simulink model "pratica_3_c"  (R2021a)
settings: Solver=VariableStepAuto  StartTime=0.0  StopTime=2  RelTol=1e-3
undefined symbols (not defined in the file): DiscIntNeverNeededParam
settings Model: Creator=ribeiro  LastModifiedBy=ribeiro

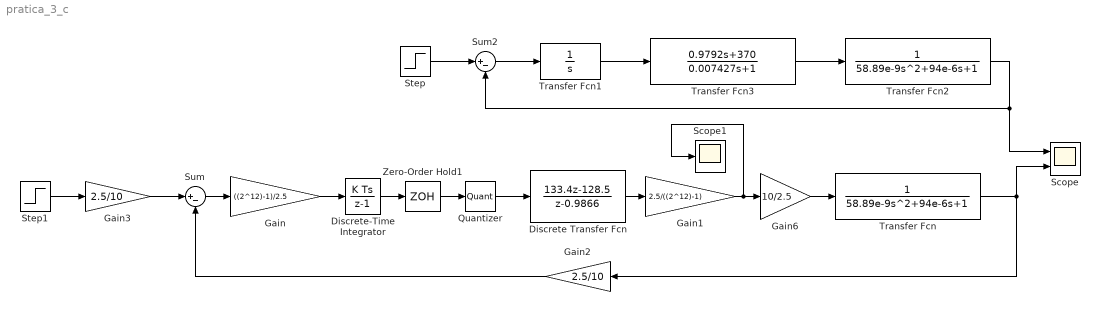
== system pratica_3_c ==
  Discrete Transfer Fcn : DiscreteTransferFcn  Numerator=[133.4 -128.5]  Denominator=[1 -0.9866]
  Discrete-Time Integrator : DiscreteIntegrator  SampleTime=-1  ICPrevOutput=DiscIntNeverNeededParam  ICPrevScaledInput=DiscIntNeverNeededParam
  Gain : Gain  Gain=((2^12)-1)/2.5
  Gain1 : Gain  Gain=2.5/((2^12)-1)
  Gain2 : Gain  Gain=2.5/10
  Gain3 : Gain  Gain=2.5/10
  Gain6 : Gain  Gain=10/2.5
  Quantizer : Quantizer  QuantizationInterval=1/((2^12)-1)
  Scope : Scope  NumInputPorts=2
  Scope1 : Scope
  Step : Step  After=10  SampleTime=0
  Step1 : Step  After=10  SampleTime=0
  Sum : Sum  Inputs=|+-
  Sum2 : Sum  Inputs=|+-
  Transfer Fcn : TransferFcn  Denominator=[58.89e-9 94e-6 1]
  Transfer Fcn1 : TransferFcn  Denominator=[1 0]
  Transfer Fcn2 : TransferFcn  Denominator=[58.89e-9 94e-6 1]
  Transfer Fcn3 : TransferFcn  Numerator=[0.9792 370]  Denominator=[0.007427 1]
  Zero-Order Hold1 : ZeroOrderHold  SampleTime=1/10000
  wires:
  Zero-Order Hold1/1 -> Quantizer/1
  Gain1/1 -> Scope1/1, Gain6/1
  Discrete Transfer Fcn/1 -> Gain1/1
  Gain6/1 -> Transfer Fcn/1
  Transfer Fcn/1 -> Gain2/1, Scope/2
  Sum/1 -> Gain/1
  Transfer Fcn3/1 -> Transfer Fcn2/1
  Transfer Fcn2/1 -> Scope/1, Sum2/2
  Step/1 -> Sum2/1
  Transfer Fcn1/1 -> Transfer Fcn3/1
  Sum2/1 -> Transfer Fcn1/1
  Gain/1 -> Discrete-Time Integrator/1
  Discrete-Time Integrator/1 -> Zero-Order Hold1/1
  Quantizer/1 -> Discrete Transfer Fcn/1
  Gain2/1 -> Sum/2
  Gain3/1 -> Sum/1
  Step1/1 -> Gain3/1
